simulink library "simscapeMultibodyLibrary"  (R2024b)
settings: Solver=VariableStepAuto  StartTime=0.0  StopTime=10.0  RelTol=1e-3
undefined symbols (not defined in the file): simscape, X, Y, Z
libraries: sm_lib x41, $bdroot x30, nesl_utility x2
settings Model: Creator=The MathWorks, Inc.  LastModifiedBy=lnicolet
settings SolverCC: AlgebraicLoopSolver=TrustRegion  MaxZcPerStep=1
settings DataIOCC: ReturnWorkspaceOutputs=off
settings OptimizationCC: LifeSpan=inf
settings DebuggingCC: UnconnectedInputMsg=warning  UnconnectedOutputMsg=warning  UnconnectedLineMsg=warning  SubsystemReferenceDiagnosticForUnitTest=warning  SFExecutionAtInitializationDiag=none  ArithmeticOperatorsInVariantConditions=warning
settings ModelReferenceCC: EnableRefExpFcnMdlSchedulingChecks=on
settings SFSimCC: CustomCodeUndefinedFunction=UseInterfaceOnly
settings RTWCC: GPUComputeCapability=3.5  DLArmComputeVersion=19.05
settings CodeAppCC: StateflowObjectComments=on

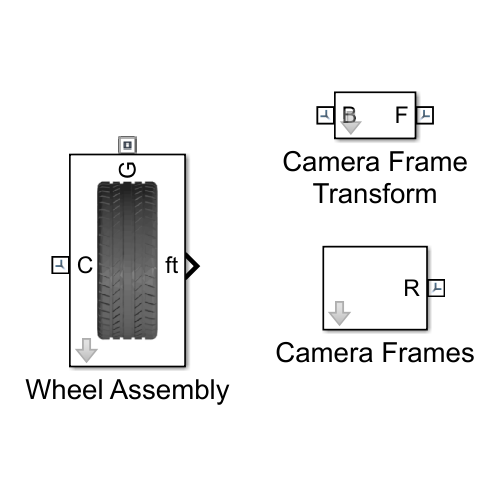
[thumbnail: Simulink's stored preview of the top-level diagram]
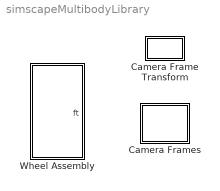
== system simscapeMultibodyLibrary ==
  Camera Frame Transform : Subsystem  mask(Define Camera Frame){CameraFrame=[]}
      mask prompts: CameraFrame "Camera Frame Data (structure)"
      mask help: Sets frame position and orientation for camera frame. Data structure provides cartesian location and orientation. Orientation is intrinsic rotation of yaw-pitch-roll.
  Camera Frames : Subsystem  mask(Camera Frames){Cameras=[]}
      mask prompts: Cameras "Cameras (structure)"
      mask help: Defines a set of frames surrounding the car for camera definition. The frames are used to define visualization viewpoints for animation of simulation results.
  Wheel Assembly : Subsystem  mask(Wheel Assembly){tire_side=Left, tire_param=simscape.multibody.tirread(''), wheel_mass=10, wheel_inertia=[1 2]}
      mask prompts: tire_side "Tire Side"; tire_param "Tire Parameters (structure)"; wheel_mass "Wheel Mass (kg)"; wheel_inertia "Wheel Inertia [Ixx Iyy] (kg*m^2)"
      mask help:
      | This block models a wheel assembly of the car. The block comprises one wheel and one tire.
      |
      | Port C corresponds to the center of the assembly with the z-axis aligned with the wheel axis.
      mask init:
      | tireSide = get_param(gcb,'tire_side');
      | set_param([gcb '/Magic Formula Tire Force and Torque'],'TireSide',tireSide);
      | 
      | sideSign = 0;
      | if(strcmpi(tireSide,'right'))
      |     sideSign = 1;
      | end
      | 
      | tire_mass = tire_param.INERTIA.MASS;
      | tire_Ixx  = tire_param.INERTIA.IXX;
      | tire_Iyy  = tire_param.INERTIA.IYY;
      | 
      | wheelAssm_mass = wheel_mass + tire_mass;
      | wheelAssm_Ixx  = wheel_inertia(1) + tire_Ixx;
      | wheelAssm_Iyy  = wheel_inertia(2) + tire_Iyy;
      | wheelAssm_I    = [wheelAssm_Ixx; wheelAssm_Iyy; wheelAssm_Ixx];
      settings: PortSchema="{\"entries\":[{\"content\":{\"sides\":[{\"content\":{\"connectorIds\":[\"LConn1\"]},\"type\":\"ConnectorPlacement.EquallySpacedRectSide\",\"uuid\":\"21c97f86-23c7-4a9b-8edb-231f5083b187\"},{\"content\":{\"connectorIds\":[\"Out1\"],\"side\":\"RIGHT\"},\"type\":\"ConnectorPlacement.EquallySpacedRectSide\",\"uuid\":\"0cc520b8-39e8-4760-b97e-e9ae4865d3f8\"},{\"content\":{\"connectorIds\":[],\"side\":\"TOP\"},\"type\":\"ConnectorPlacement.EquallySpacedRectSide\",\"uuid\":\"60676e24-b348-4ad9-acd0-dd2f876ae5f6\"},{\"content\":{\"connectorIds\":[\"RConn1\"],\"side\":\"BOTTOM\"},\"type\":\"ConnectorPlacement.EquallySpacedRectSide\",\"uuid\":\"e7cf26ce-1721-48f1-8ffe-031fa37b7827\"}]},\"type\":\"ConnectorPlacement.EquallySpacedConnector\",\"uuid\":\"13eec707-bcd2-4a1c-b172-275fe00d8ff3\"}],\"packageUris\":[\"http://schema.mathworks.com/mf0/Connector/R2020b\"],\"version\":\"1.0\"}"
      mask TypeOptions tire_side: Left | Right
      mask Display: image('Wheel.png')

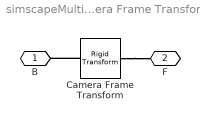
== system simscapeMultibodyLibrary/Camera Frame Transform ==
  Camera Frame Transform : sm_lib/Frames and Transforms/Rigid Transform  RotationMethod=RotationSequence  FollAlignAxisA=+X  BaseAlignAxisA=+Y  FollAlignAxisB=+Y  BaseAlignAxisB=+Z  RotationStandardAxis=+Z  RotationAngle=0.0  RotationAngleUnits=deg  RotationArbitraryAxis=[0 0 1]  RotationSequenceAxes=FollowerAxes  RotationSequence=ZYX  RotationSequenceAngles=CameraFrame.a.Value(3:-1:1)  RotationSequenceAnglesUnits=deg  RotationMatrix=[1 0 0; 0 1 0; 0 0 1]  Quaternion=[1 0 0 0]  TranslationMethod=Cartesian  TranslationCartesianOffset=CameraFrame.s.Value  TranslationCartesianOffsetUnits=m  TranslationStandardAxis=+Z  TranslationStandardOffset=0  TranslationStandardOffsetUnits=m  TranslationROffset=0  TranslationROffsetUnits=m  TranslationThetaOffset=0  TranslationThetaOffsetUnits=deg  TranslationZOffset=0  TranslationZOffsetUnits=m
  B : PMIOPort  Side=Left
  F : PMIOPort  Port=2  Side=Right
  connections:
  Camera Frame Transform/LConn1 -- B/RConn1
  Camera Frame Transform/RConn1 -- F/RConn1

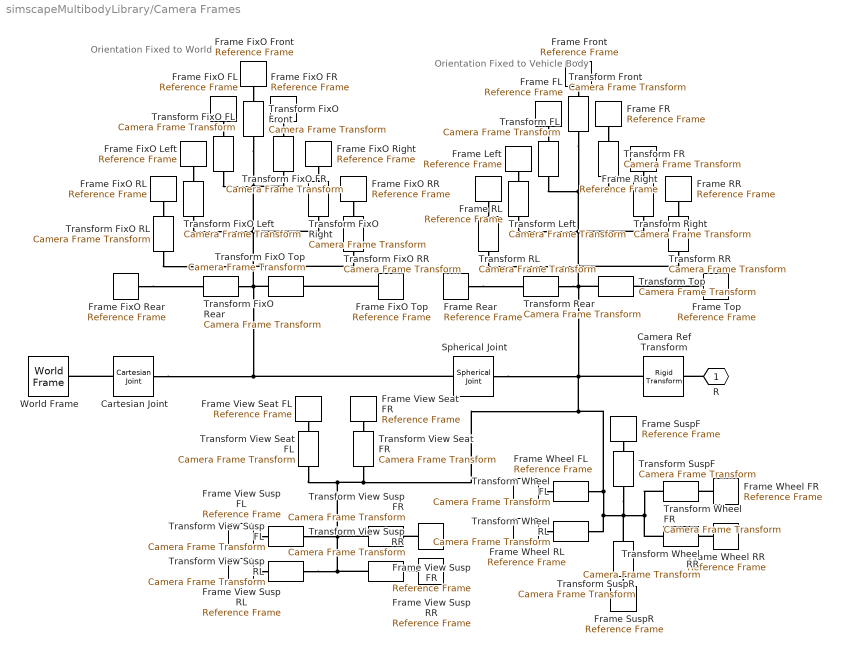
== system simscapeMultibodyLibrary/Camera Frames ==
  note: Orientation Fixed to Vehicle Body
  note: Orientation Fixed to World
  Camera Ref Transform : sm_lib/Frames and Transforms/Rigid Transform  RotationMethod=RotationSequence  FollAlignAxisA=+X  BaseAlignAxisA=+Y  FollAlignAxisB=+Y  BaseAlignAxisB=+Z  RotationStandardAxis=+Z  RotationAngle=0.0  RotationAngleUnits=deg  RotationArbitraryAxis=[0 0 1]  RotationSequenceAxes=FollowerAxes  RotationSequence=ZYX  RotationSequenceAngles=[Cameras.Offset.a.Value(3) Cameras.Offset.a.Value(2) Cameras.Offset.a.Value(1)]  RotationSequenceAnglesUnits=deg  RotationMatrix=[1 0 0; 0 1 0; 0 0 1]  Quaternion=[1 0 0 0]  TranslationMethod=Cartesian  TranslationCartesianOffset=Cameras.Offset.s.Value  TranslationCartesianOffsetUnits=m  TranslationStandardAxis=+Z  TranslationStandardOffset=0  TranslationStandardOffsetUnits=m  TranslationROffset=0  TranslationROffsetUnits=m  TranslationThetaOffset=0  TranslationThetaOffsetUnits=deg  TranslationZOffset=0  TranslationZOffsetUnits=m
  Cartesian Joint : sm_lib/Joints/Cartesian Joint  JointMode=Normal  CompositeWrenchDir=FollowerOnBase  CompositeWrenchFrame=BaseFrame  SenseConstraintForce=off  SenseConstraintTorque=off  SenseTotalForce=off  SenseTotalTorque=off  PxPositionTargetSpecify=off  PxPositionTargetPriority=High  PxPositionTargetValue=0  PxPositionTargetValueUnits=m  PxVelocityTargetSpecify=off  PxVelocityTargetPriority=High  PxVelocityTargetValue=0  PxVelocityTargetValueUnits=m/s  PxEquilibriumPosition=0  PxEquilibriumPositionUnits=m  PxSpringStiffness=0  PxSpringStiffnessUnits=N/m  PxDampingCoefficient=0  PxDampingCoefficientUnits=N/(m/s)  PxLowerLimitSpecify=off  PxLowerLimitBound=-1  PxLowerLimitBoundUnits=m  PxLowerLimitStiffness=1e6  PxLowerLimitStiffnessUnits=N/m  PxLowerLimitDamping=1e3  PxLowerLimitDampingUnits=N/(m/s)  PxLowerLimitTransitionRegionWidth=1e-4  PxLowerLimitTransitionRegionWidthUnits=m  PxUpperLimitSpecify=off  PxUpperLimitBound=1  PxUpperLimitBoundUnits=m  PxUpperLimitStiffness=1e6  PxUpperLimitStiffnessUnits=N/m  PxUpperLimitDamping=1e3  PxUpperLimitDampingUnits=N/(m/s)  PxUpperLimitTransitionRegionWidth=1e-4  PxUpperLimitTransitionRegionWidthUnits=m  PxTorqueActuationMode=NoTorque  PxMotionActuationMode=ComputedMotion  PxSensePosition=off  PxSenseVelocity=off  PxSenseAcceleration=off  PxSenseTorqueForce=off  PxSenseLowerLimitTorqueForce=off  PxSenseUpperLimitTorqueForce=off  PyPositionTargetSpecify=off  PyPositionTargetPriority=High  PyPositionTargetValue=0  PyPositionTargetValueUnits=m  PyVelocityTargetSpecify=off  PyVelocityTargetPriority=High  PyVelocityTargetValue=0  PyVelocityTargetValueUnits=m/s  PyEquilibriumPosition=0  PyEquilibriumPositionUnits=m  PySpringStiffness=0  PySpringStiffnessUnits=N/m  PyDampingCoefficient=0  PyDampingCoefficientUnits=N/(m/s)  PyLowerLimitSpecify=off  PyLowerLimitBound=-1  PyLowerLimitBoundUnits=m  PyLowerLimitStiffness=1e6  PyLowerLimitStiffnessUnits=N/m  PyLowerLimitDamping=1e3  PyLowerLimitDampingUnits=N/(m/s)  PyLowerLimitTransitionRegionWidth=1e-4  PyLowerLimitTransitionRegionWidthUnits=m  PyUpperLimitSpecify=off  PyUpperLimitBound=1  PyUpperLimitBoundUnits=m  PyUpperLimitStiffness=1e6  PyUpperLimitStiffnessUnits=N/m  PyUpperLimitDamping=1e3  PyUpperLimitDampingUnits=N/(m/s)  PyUpperLimitTransitionRegionWidth=1e-4  PyUpperLimitTransitionRegionWidthUnits=m  PyTorqueActuationMode=NoTorque  PyMotionActuationMode=ComputedMotion  PySensePosition=off  PySenseVelocity=off  PySenseAcceleration=off  PySenseTorqueForce=off  PySenseLowerLimitTorqueForce=off  PySenseUpperLimitTorqueForce=off  PzPositionTargetSpecify=off  PzPositionTargetPriority=High  PzPositionTargetValue=0  PzPositionTargetValueUnits=m  PzVelocityTargetSpecify=off  PzVelocityTargetPriority=High  PzVelocityTargetValue=0  PzVelocityTargetValueUnits=m/s  PzEquilibriumPosition=0  PzEquilibriumPositionUnits=m  PzSpringStiffness=0  PzSpringStiffnessUnits=N/m  PzDampingCoefficient=0  PzDampingCoefficientUnits=N/(m/s)  PzLowerLimitSpecify=off  PzLowerLimitBound=-1  PzLowerLimitBoundUnits=m  PzLowerLimitStiffness=1e6  PzLowerLimitStiffnessUnits=N/m  PzLowerLimitDamping=1e3  PzLowerLimitDampingUnits=N/(m/s)  PzLowerLimitTransitionRegionWidth=1e-4  PzLowerLimitTransitionRegionWidthUnits=m  PzUpperLimitSpecify=off  PzUpperLimitBound=1  PzUpperLimitBoundUnits=m  PzUpperLimitStiffness=1e6  PzUpperLimitStiffnessUnits=N/m  PzUpperLimitDamping=1e3  PzUpperLimitDampingUnits=N/(m/s)  PzUpperLimitTransitionRegionWidth=1e-4  PzUpperLimitTransitionRegionWidthUnits=m  PzTorqueActuationMode=NoTorque  PzMotionActuationMode=ComputedMotion  PzSensePosition=off  PzSenseVelocity=off  PzSenseAcceleration=off  PzSenseTorqueForce=off  PzSenseLowerLimitTorqueForce=off  PzSenseUpperLimitTorqueForce=off
  Frame FL : sm_lib/Frames and Transforms/Reference Frame
  Frame FR : sm_lib/Frames and Transforms/Reference Frame
  Frame FixO FL : sm_lib/Frames and Transforms/Reference Frame
  Frame FixO FR : sm_lib/Frames and Transforms/Reference Frame
  Frame FixO Front : sm_lib/Frames and Transforms/Reference Frame
  Frame FixO Left : sm_lib/Frames and Transforms/Reference Frame
  Frame FixO RL : sm_lib/Frames and Transforms/Reference Frame
  Frame FixO RR : sm_lib/Frames and Transforms/Reference Frame
  Frame FixO Rear : sm_lib/Frames and Transforms/Reference Frame
  Frame FixO Right : sm_lib/Frames and Transforms/Reference Frame
  Frame FixO Top : sm_lib/Frames and Transforms/Reference Frame
  Frame Front : sm_lib/Frames and Transforms/Reference Frame
  Frame Left : sm_lib/Frames and Transforms/Reference Frame
  Frame RL : sm_lib/Frames and Transforms/Reference Frame
  Frame RR : sm_lib/Frames and Transforms/Reference Frame
  Frame Rear : sm_lib/Frames and Transforms/Reference Frame
  Frame Right : sm_lib/Frames and Transforms/Reference Frame
  Frame SuspF : sm_lib/Frames and Transforms/Reference Frame
  Frame SuspR : sm_lib/Frames and Transforms/Reference Frame
  Frame Top : sm_lib/Frames and Transforms/Reference Frame
  Frame View Seat FL : sm_lib/Frames and Transforms/Reference Frame
  Frame View Seat FR : sm_lib/Frames and Transforms/Reference Frame
  Frame View Susp FL : sm_lib/Frames and Transforms/Reference Frame
  Frame View Susp FR : sm_lib/Frames and Transforms/Reference Frame
  Frame View Susp RL : sm_lib/Frames and Transforms/Reference Frame
  Frame View Susp RR : sm_lib/Frames and Transforms/Reference Frame
  Frame Wheel FL : sm_lib/Frames and Transforms/Reference Frame
  Frame Wheel FR : sm_lib/Frames and Transforms/Reference Frame
  Frame Wheel RL : sm_lib/Frames and Transforms/Reference Frame
  Frame Wheel RR : sm_lib/Frames and Transforms/Reference Frame
  Spherical Joint : sm_lib/Joints/Spherical Joint  JointMode=Normal  CompositeWrenchDir=FollowerOnBase  CompositeWrenchFrame=BaseFrame  SenseConstraintForce=off  SenseConstraintTorque=off  SenseTotalForce=off  SenseTotalTorque=off  PositionTargetSpecify=off  PositionTargetPriority=High  PositionTargetRotationMethod=None  PositionTargetFollAlignAxisA=+X  PositionTargetBaseAlignAxisA=+Y  PositionTargetFollAlignAxisB=+Y  PositionTargetBaseAlignAxisB=+Z  PositionTargetRotationStandardAxis=+Z  PositionTargetRotationAngle=0.0  PositionTargetRotationAngleUnits=deg  PositionTargetRotationArbitraryAxis=[0 0 1]  PositionTargetRotationSequenceAxes=FollowerAxes  PositionTargetRotationSequence=XYX  PositionTargetRotationSequenceAngles=[0 0 0]  PositionTargetRotationSequenceAnglesUnits=deg  PositionTargetRotationMatrix=[1 0 0; 0 1 0; 0 0 1]  PositionTargetQuaternion=[1 0 0 0]  VelocityTargetSpecify=off  VelocityTargetPriority=High  VelocityTargetValue=[0 0 0]  VelocityTargetValueUnits=deg/s  VelocityTargetInFollowerFrame=on  EqPosRotationMethod=None  EqPosFollAlignAxisA=+X  EqPosBaseAlignAxisA=+Y  EqPosFollAlignAxisB=+Y  EqPosBaseAlignAxisB=+Z  EqPosRotationStandardAxis=+Z  EqPosRotationAngle=0.0  EqPosRotationAngleUnits=deg  EqPosRotationArbitraryAxis=[0 0 1]  EqPosRotationSequenceAxes=FollowerAxes  EqPosRotationSequence=XYX  EqPosRotationSequenceAngles=[0 0 0]  EqPosRotationSequenceAnglesUnits=deg  EqPosRotationMatrix=[1 0 0; 0 1 0; 0 0 1]  EqPosQuaternion=[1 0 0 0]  SpringStiffness=0  SpringStiffnessUnits=N*m/deg  DampingCoefficient=0  DampingCoefficientUnits=N*m/(deg/s)  LowerLimitSpecify=off  LowerLimitBound=15  LowerLimitBoundUnits=deg  LowerLimitStiffness=1e4  LowerLimitStiffnessUnits=N*m/deg  LowerLimitDamping=10  LowerLimitDampingUnits=N*m/(deg/s)  LowerLimitTransitionRegionWidth=0.1  LowerLimitTransitionRegionWidthUnits=deg  UpperLimitSpecify=off  UpperLimitBound=45  UpperLimitBoundUnits=deg  UpperLimitStiffness=1e4  UpperLimitStiffnessUnits=N*m/deg  UpperLimitDamping=10  UpperLimitDampingUnits=N*m/(deg/s)  UpperLimitTransitionRegionWidth=0.1  UpperLimitTransitionRegionWidthUnits=deg  TorqueActuationMode=NoTorque  ActuateTorqueX=off  ActuateTorqueY=off  ActuateTorqueZ=off  ActuateTorque=off  ActuationFrame=BaseFrame  SensePosition=off  SenseVelocityX=off  SenseVelocityY=off  SenseVelocityZ=off  SenseVelocity=off  SenseAccelerationX=off  SenseAccelerationY=off  SenseAccelerationZ=off  SenseAcceleration=off  SenseLowerLimitTorqueMag=off  SenseUpperLimitTorqueMag=off  SensingFrame=BaseFrame
  Transform FL : $bdroot/Camera Frame Transform  CameraFrame=Cameras.FL
  Transform FR : $bdroot/Camera Frame Transform  CameraFrame=Cameras.FR
  Transform FixO FL : $bdroot/Camera Frame Transform  CameraFrame=Cameras.FL
  Transform FixO FR : $bdroot/Camera Frame Transform  CameraFrame=Cameras.FR
  Transform FixO Front : $bdroot/Camera Frame Transform  CameraFrame=Cameras.Front
  Transform FixO Left : $bdroot/Camera Frame Transform  CameraFrame=Cameras.Left
  Transform FixO RL : $bdroot/Camera Frame Transform  CameraFrame=Cameras.RL
  Transform FixO RR : $bdroot/Camera Frame Transform  CameraFrame=Cameras.RR
  Transform FixO Rear : $bdroot/Camera Frame Transform  CameraFrame=Cameras.Rear
  Transform FixO Right : $bdroot/Camera Frame Transform  CameraFrame=Cameras.Right
  Transform FixO Top : $bdroot/Camera Frame Transform  CameraFrame=Cameras.Top
  Transform Front : $bdroot/Camera Frame Transform  CameraFrame=Cameras.Front
  Transform Left : $bdroot/Camera Frame Transform  CameraFrame=Cameras.Left
  Transform RL : $bdroot/Camera Frame Transform  CameraFrame=Cameras.RL
  Transform RR : $bdroot/Camera Frame Transform  CameraFrame=Cameras.RR
  Transform Rear : $bdroot/Camera Frame Transform  CameraFrame=Cameras.Rear
  Transform Right : $bdroot/Camera Frame Transform  CameraFrame=Cameras.Right
  Transform SuspF : $bdroot/Camera Frame Transform  CameraFrame=Cameras.SuspF
  Transform SuspR : $bdroot/Camera Frame Transform  CameraFrame=Cameras.SuspR
  Transform Top : $bdroot/Camera Frame Transform  CameraFrame=Cameras.Top
  Transform View Seat FL : $bdroot/Camera Frame Transform  CameraFrame=Cameras.View_SeatFL
  Transform View Seat FR : $bdroot/Camera Frame Transform  CameraFrame=Cameras.View_SeatFR
  Transform View Susp FL : $bdroot/Camera Frame Transform  CameraFrame=Cameras.View_SuspFL
  Transform View Susp FR : $bdroot/Camera Frame Transform  CameraFrame=Cameras.View_SuspFR
  Transform View Susp RL : $bdroot/Camera Frame Transform  CameraFrame=Cameras.View_SuspRL
  Transform View Susp RR : $bdroot/Camera Frame Transform  CameraFrame=Cameras.View_SuspRR
  Transform Wheel FL : $bdroot/Camera Frame Transform  CameraFrame=Cameras.Wheel_FL
  Transform Wheel FR : $bdroot/Camera Frame Transform  CameraFrame=Cameras.Wheel_FR
  Transform Wheel RL : $bdroot/Camera Frame Transform  CameraFrame=Cameras.Wheel_RL
  Transform Wheel RR : $bdroot/Camera Frame Transform  CameraFrame=Cameras.Wheel_RR
  World Frame : sm_lib/Frames and Transforms/World Frame
  R : PMIOPort  Side=Right
  connections:
  R/RConn1 -- Camera Ref Transform/LConn1
  Transform View Susp FR/LConn1 -- Transform View Susp RL/LConn1 -- Transform View Susp RR/LConn1 -- Transform View Susp FL/LConn1 -- Transform View Seat FR/LConn1 -- Transform Wheel FL/LConn1 -- Transform Wheel RL/LConn1 -- Transform SuspR/LConn1 -- Transform SuspF/LConn1 -- Transform Wheel RR/LConn1 -- Transform Wheel FR/LConn1 -- Spherical Joint/RConn1 -- Camera Ref Transform/RConn1 -- Transform Top/LConn1 -- Transform Rear/LConn1 -- Transform RL/LConn1 -- Transform RR/LConn1 -- Transform Left/LConn1 -- Transform Right/LConn1 -- Transform FR/LConn1 -- Transform Front/LConn1 -- Transform FL/LConn1 -- Transform View Seat FL/LConn1
  Cartesian Joint/LConn1 -- World Frame/RConn1
  Cartesian Joint/RConn1 -- Spherical Joint/LConn1 -- Transform FixO Rear/LConn1 -- Transform FixO Top/LConn1 -- Transform FixO RR/LConn1 -- Transform FixO RL/LConn1 -- Transform FixO Right/LConn1 -- Transform FixO Left/LConn1 -- Transform FixO FL/LConn1 -- Transform FixO Front/LConn1 -- Transform FixO FR/LConn1
  Frame FixO FR/RConn1 -- Transform FixO FR/RConn1
  Frame FixO Right/RConn1 -- Transform FixO Right/RConn1
  Frame FixO RR/RConn1 -- Transform FixO RR/RConn1
  Frame FixO RL/RConn1 -- Transform FixO RL/RConn1
  Frame FixO Left/RConn1 -- Transform FixO Left/RConn1
  Frame FixO FL/RConn1 -- Transform FixO FL/RConn1
  Frame FixO Top/RConn1 -- Transform FixO Top/RConn1
  Frame FixO Front/RConn1 -- Transform FixO Front/RConn1
  Frame FixO Rear/RConn1 -- Transform FixO Rear/RConn1
  Frame Rear/RConn1 -- Transform Rear/RConn1
  Frame Top/RConn1 -- Transform Top/RConn1
  Frame Left/RConn1 -- Transform Left/RConn1
  Frame FL/RConn1 -- Transform FL/RConn1
  Frame RL/RConn1 -- Transform RL/RConn1
  Frame Right/RConn1 -- Transform Right/RConn1
  Frame FR/RConn1 -- Transform FR/RConn1
  Frame RR/RConn1 -- Transform RR/RConn1
  Frame Front/RConn1 -- Transform Front/RConn1
  Frame SuspF/RConn1 -- Transform SuspF/RConn1
  Frame SuspR/RConn1 -- Transform SuspR/RConn1
  Frame Wheel FR/RConn1 -- Transform Wheel FR/RConn1
  Frame Wheel RR/RConn1 -- Transform Wheel RR/RConn1
  Frame Wheel FL/RConn1 -- Transform Wheel FL/RConn1
  Frame Wheel RL/RConn1 -- Transform Wheel RL/RConn1
  Frame View Seat FL/RConn1 -- Transform View Seat FL/RConn1
  Frame View Seat FR/RConn1 -- Transform View Seat FR/RConn1
  Frame View Susp FL/RConn1 -- Transform View Susp FL/RConn1
  Frame View Susp FR/RConn1 -- Transform View Susp FR/RConn1
  Frame View Susp RR/RConn1 -- Transform View Susp RR/RConn1
  Frame View Susp RL/RConn1 -- Transform View Susp RL/RConn1

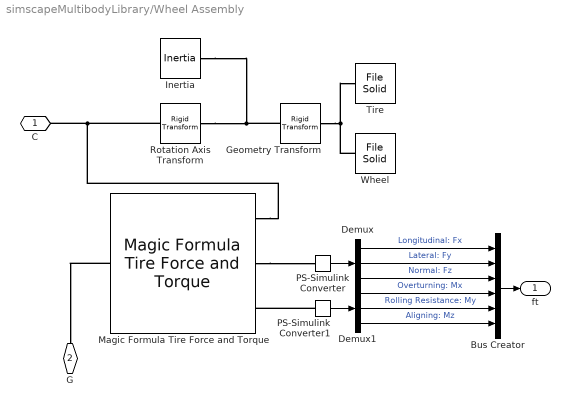
== system simscapeMultibodyLibrary/Wheel Assembly ==
  Bus Creator : BusCreator  Inputs=6
  Demux : Demux  Outputs=3
  Demux1 : Demux  Outputs=3
  Geometry Transform : sm_lib/Frames and Transforms/Rigid Transform  RotationMethod=StandardAxis  FollAlignAxisA=+X  BaseAlignAxisA=+Y  FollAlignAxisB=+Y  BaseAlignAxisB=+Z  RotationStandardAxis=+X  RotationAngle=sideSign*180-90  RotationAngleUnits=deg  RotationArbitraryAxis=[0 0 1]  RotationSequenceAxes=FollowerAxes  RotationSequence=XYX  RotationSequenceAngles=[0 0 0]  RotationSequenceAnglesUnits=deg  RotationMatrix=[1 0 0; 0 1 0; 0 0 1]  Quaternion=[1 0 0 0]  TranslationMethod=StandardAxis  TranslationCartesianOffset=[0 0 0]  TranslationCartesianOffsetUnits=m  TranslationStandardAxis=+Y  TranslationStandardOffset=(1-2*sideSign)*0.125  TranslationStandardOffsetUnits=m  TranslationROffset=0  TranslationROffsetUnits=m  TranslationThetaOffset=0  TranslationThetaOffsetUnits=deg  TranslationZOffset=0  TranslationZOffsetUnits=m
  Inertia : sm_lib/Body Elements/Inertia  InertiaType=Custom  Mass=wheelAssm_mass  MassUnits=kg  CenterOfMass=[0 0 0]  CenterOfMassUnits=m  MomentsOfInertia=wheelAssm_I  MomentsOfInertiaUnits=kg*m^2  ProductsOfInertia=[0 0 0]  ProductsOfInertiaUnits=kg*m^2  GraphicType=None  MarkerShape=Inertia  MarkerSize=20  GraphicVisPropType=SimpleVisualProperties  GraphicDiffuseColor=[0.5 0.5 0.5]  GraphicOpacity=1.0  GraphicSpecularColor=[0.5 0.5 0.5 1.0]  GraphicAmbientColor=[0.15 0.15 0.15 1.0]  GraphicEmissiveColor=[0.0 0.0 0.0 1.0]  GraphicShininess=75
  Magic Formula Tire Force and Torque : sm_lib/Forces and Torques/Magic Formula Tire Force and Torque  TireSide=Left  TireParameters=tire_param  SlipMode=Combined  ContactFrameMethod=ClosestPoint  ScalingCoefficientLMUXMode=FromTireParameters  ScalingCoefficientLMUYMode=FromTireParameters  SenseContactSignal=off  TireWrenchFrame=ContactFrame  SenseTireForce=on  SenseTireTorque=on  SensePneumaticTrail=off  SenseLongitudinalSlip=off  SenseSaturatedLongitudinalSlip=off  SenseSlipAngle=off  SenseSaturatedSlipAngle=off  SenseTurnSlip=off  SenseRelativeLongitudinalVelocity=off  SenseRelativeLateralVelocity=off  SenseLongitudinalSlipVelocity=off  SenseLateralSlipVelocity=off  SenseYawVelocity=off  SenseCamberAngle=off  SenseSaturatedCamberAngle=off  SenseCamberVelocity=off  SenseSpinVelocity=off  SenseFreeRadius=off  SenseLoadedRadius=off  SenseEffectiveRollingRadius=off  SenseRadialDeflection=off  SenseLongitudinalFrictionCoefficient=off  SenseLateralFrictionCoefficient=off  SenseContactBaseRotation=off  SenseContactBaseTranslation=off  SenseContactFollowerRotation=off  SenseContactFollowerTranslation=off  NumericParameters=[0.1 0.1 0.1 0.1 0.1 1e-4 1e-4 1e-7 1e-7 1e-4 1e-4 0.1 1e-4 1e-4 1e-4 1e-4 1e-4 1e-4 1e-4 1e-4 1e-4]
  PS-Simulink Converter : nesl_utility/PS-Simulink Converter  PhysicalDomain=network_engine_domain  SubClassName=ps_output  LeftPortType=input  RightPortType=output  PseudoPeriodic=off  Frequencies=[]  VectorFormat=1-D array  Unit=inherit  AffineConversion=off
  PS-Simulink Converter1 : nesl_utility/PS-Simulink Converter  PhysicalDomain=network_engine_domain  SubClassName=ps_output  LeftPortType=input  RightPortType=output  PseudoPeriodic=off  Frequencies=[]  VectorFormat=1-D array  Unit=inherit  AffineConversion=off
  Rotation Axis Transform : sm_lib/Frames and Transforms/Rigid Transform  RotationMethod=AlignedAxes  FollAlignAxisA=+X  BaseAlignAxisA=+X  FollAlignAxisB=+Z  BaseAlignAxisB=+Y  RotationStandardAxis=-X  RotationAngle=0  RotationAngleUnits=deg  RotationArbitraryAxis=[0 0 1]  RotationSequenceAxes=FollowerAxes  RotationSequence=XYX  RotationSequenceAngles=[0 0 0]  RotationSequenceAnglesUnits=deg  RotationMatrix=[1 0 0; 0 1 0; 0 0 1]  Quaternion=[1 0 0 0]  TranslationMethod=None  TranslationCartesianOffset=[0 0 0]  TranslationCartesianOffsetUnits=m  TranslationStandardAxis=+Z  TranslationStandardOffset=0  TranslationStandardOffsetUnits=m  TranslationROffset=0  TranslationROffsetUnits=m  TranslationThetaOffset=0  TranslationThetaOffsetUnits=deg  TranslationZOffset=0  TranslationZOffsetUnits=m
  Tire : sm_lib/Body Elements/File Solid  ExtGeomFileName=Tire.STL  UnitType=Custom  ExtGeomFileUnits=mm  StepReaderType=HEX  ExportConvexHullGeometry=off  InertiaType=Custom  BasedOnType=Density  Density=1000  DensityUnits=kg/m^3  Mass=0  MassUnits=kg  CenterOfMass=[0 0 0]  CenterOfMassUnits=m  MomentsOfInertia=[0 0 0]  MomentsOfInertiaUnits=kg*m^2  ProductsOfInertia=[0 0 0]  ProductsOfInertiaUnits=kg*m^2  GraphicType=FromGeometry  MarkerShape=Sphere  MarkerSize=10  GraphicVisPropType=SimpleVisualProperties  GraphicDiffuseColor=[0.5 0.5 0.5]  GraphicOpacity=1.0  GraphicSpecularColor=[0.5 0.5 0.5 1.0]  GraphicAmbientColor=[0.15 0.15 0.15 1.0]  GraphicEmissiveColor=[0.0 0.0 0.0 1.0]  GraphicShininess=75  DoExposeReferenceFrame=on  SerializedFrames=<Frames/>
  Wheel : sm_lib/Body Elements/File Solid  ExtGeomFileName=Wheel.STL  UnitType=Custom  ExtGeomFileUnits=mm  StepReaderType=HEX  ExportConvexHullGeometry=off  InertiaType=Custom  BasedOnType=Density  Density=1000  DensityUnits=kg/m^3  Mass=0  MassUnits=kg  CenterOfMass=[0 0 0]  CenterOfMassUnits=m  MomentsOfInertia=[0 0 0]  MomentsOfInertiaUnits=kg*m^2  ProductsOfInertia=[0 0 0]  ProductsOfInertiaUnits=kg*m^2  GraphicType=FromGeometry  MarkerShape=Sphere  MarkerSize=10  GraphicVisPropType=SimpleVisualProperties  GraphicDiffuseColor=[0.8 0.8 0.8]  GraphicOpacity=1.0  GraphicSpecularColor=[0.5 0.5 0.5 1.0]  GraphicAmbientColor=[0.15 0.15 0.15 1.0]  GraphicEmissiveColor=[0.0 0.0 0.0 1.0]  GraphicShininess=75  DoExposeReferenceFrame=on  SerializedFrames=<Frames/>
  C : PMIOPort  Side=Left
  G : PMIOPort  Port=2  Side=Right
  ft : Outport
  wires:
  PS-Simulink Converter/1 -> Demux/1
  Demux/1 -> Bus Creator/1  "Longitudinal: Fx"
  Demux/2 -> Bus Creator/2  "Lateral: Fy"
  Demux/3 -> Bus Creator/3  "Normal: Fz"
  Demux1/3 -> Bus Creator/6  "Aligning: Mz"
  Demux1/2 -> Bus Creator/5  "Rolling Resistance: My"
  Demux1/1 -> Bus Creator/4  "Overturning: Mx"
  PS-Simulink Converter1/1 -> Demux1/1
  Bus Creator/1 -> ft/1
  connections:
  Wheel/RConn1 -- Geometry Transform/RConn1 -- Tire/RConn1
  Inertia/RConn1 -- Geometry Transform/LConn1 -- Rotation Axis Transform/LConn1
  Magic Formula Tire Force and Torque/LConn1 -- G/RConn1
  Magic Formula Tire Force and Torque/RConn2 -- PS-Simulink Converter/LConn1
  PS-Simulink Converter1/LConn1 -- Magic Formula Tire Force and Torque/RConn3
  Rotation Axis Transform/RConn1 -- Magic Formula Tire Force and Torque/RConn1 -- C/RConn1
